simulink subsystem "PI_original"  (R2020b)
settings: Solver=VariableStepAuto  StartTime=0.0  StopTime=10.0  RelTol=1e-3
values from neighbouring files (symbols this model uses):
  Gamma12_z = -0.308384893038560    (= -0.308384893039)    [PI_original_parameters.m]
  Gamma21_z = -0.829434052560960    (= -0.829434052561)    [PI_original_parameters.m]
  K_P_11 = 1.653001431483017    (= 1.65300143148)    [PI_original_parameters.m]
  K_P_22 = 4.162509742530150    (= 4.16250974253)    [PI_original_parameters.m]
  T_I_11 = 841.6941455268073    (= 841.694145527)    [PI_original_parameters.m]
  T_I_22 = 757.1049307125121    (= 757.104930713)    [PI_original_parameters.m]
  zone_1_ctrl_idx = 5    [PI_original_parameters.m]
  zone_2_ctrl_idx = 10    [PI_original_parameters.m]
undefined symbols (not defined in the file or in its folder): T_c
settings Model: Creator=leop9  LastModifiedBy=Previ

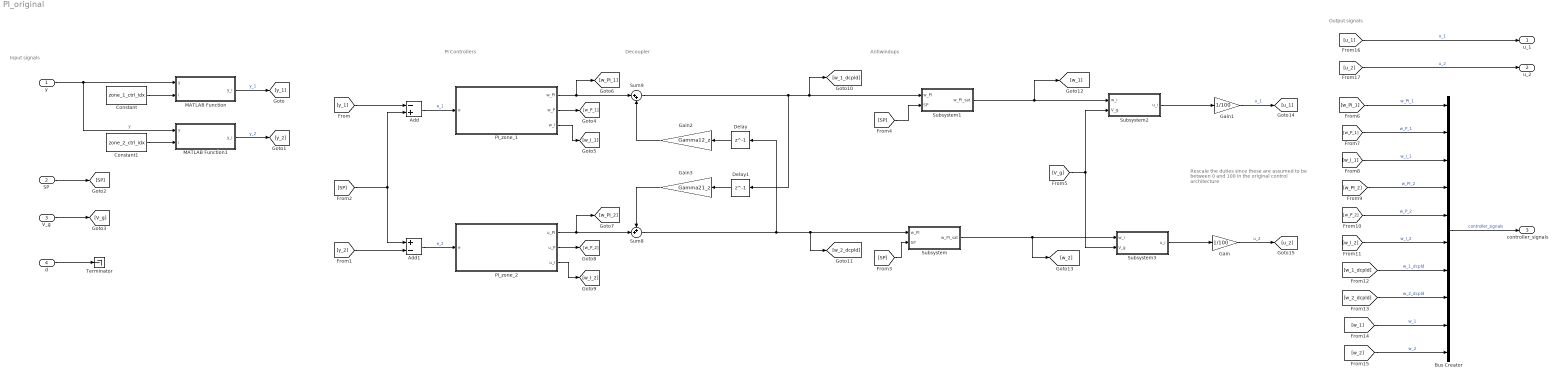
== system PI_original ==
  note: Output signals
  note: Antiwindups
  note: Decoupler
  note: Rescale the duties since these are assumed to be between 0 and 100 in the original control architecture
  note: PI Controllers
  note: Input signals
  y : Inport
  SP : Inport  Port=2
  V_g : Inport  Port=3
  d : Inport  Port=4
  Add : Sum  Inputs=-+
  Add1 : Sum  Inputs=+-
  Bus Creator : BusCreator  Inputs=10
  Constant : Constant  Value=zone_1_ctrl_idx
  Constant1 : Constant  Value=zone_2_ctrl_idx
  Delay : Delay  DelayLength=1  InitialCondition=0  SampleTime=T_c
  Delay1 : Delay  DelayLength=1  InitialCondition=0  SampleTime=T_c
  Gain : Gain  Gain=1/100
  Gain1 : Gain  Gain=1/100
  Gain2 : Gain  Gain=Gamma12_z
  Gain3 : Gain  Gain=Gamma21_z
  MATLAB Function : MATLAB Function  TreatAsAtomicUnit=on
  MATLAB Function1 : MATLAB Function  TreatAsAtomicUnit=on
  PI_zone_1 : Subsystem
  PI_zone_2 : Subsystem
  Subsystem : Subsystem
  Subsystem1 : Subsystem
  Subsystem2 : Subsystem
  Subsystem3 : Subsystem
  Sum8 : Sum  Inputs=++|
  Sum9 : Sum  Inputs=|++
  Terminator : Terminator
  u_1 : Outport
  u_2 : Outport  Port=2
  controller_signals : Outport  Port=3
  wires:
  Bus Creator/1 -> controller_signals/1  "controller_signals"
  [u_2] -> u_2/1  "u_2"
  [u_1] -> u_1/1  "u_1"
  [w_2] -> Bus Creator/10  "w_2"
  [w_1] -> Bus Creator/9  "w_1"
  [w_2_dcpld] -> Bus Creator/8  "w_2_dcpld"
  [w_1_dcpld] -> Bus Creator/7  "w_1_dcpld"
  [w_I_2] -> Bus Creator/6  "w_I_2"
  [w_P_2] -> Bus Creator/5  "w_P_2"
  [w_PI_2] -> Bus Creator/4  "w_PI_2"
  [w_I_1] -> Bus Creator/3  "w_I_1"
  [w_P_1] -> Bus Creator/2  "w_P_1"
  [w_PI_1] -> Bus Creator/1  "w_PI_1"
  PI_zone_2/3(u_I) -> [w_I_2]
  PI_zone_2/2(u_P) -> [w_P_2]
  PI_zone_1/3(w_I) -> [w_I_1]
  PI_zone_1/2(w_P) -> [w_P_1]
  [SP] -> Subsystem1/2(SP)
  [SP] -> Subsystem/2(SP)
  d/1 -> Terminator/1
  V_g/1 -> [V_g]
  SP/1 -> [SP]
  Constant1/1 -> MATLAB Function1/2(i)
  MATLAB Function1/1(y_i) -> [y_2]  "y_2"
  MATLAB Function/1(y_i) -> [y_1]  "y_1"
  Constant/1 -> MATLAB Function/2(i)
  y/1 -> MATLAB Function1/1(y), MATLAB Function/1(y)  "y"
  [y_2] -> Add1/2
  [y_1] -> Add/1
  Gain/1 -> [u_2]  "u_2"
  Gain1/1 -> [u_1]  "u_1"
  Subsystem2/1(u_i) -> Gain1/1
  Subsystem1/1(w_PI_sat) -> [w_1], Subsystem2/1(w_i)
  Subsystem3/1(u_i) -> Gain/1
  [V_g] -> Subsystem3/2(V_g), Subsystem2/2(V_g)
  [SP] -> Add1/1, Add/2
  Gain3/1 -> Sum8/1
  Add/1 -> PI_zone_1/1(e)  "e_1"
  Add1/1 -> PI_zone_2/1(e)  "e_2"
  Sum8/1 -> [w_2_dcpld], Subsystem/1(w_PI), Delay/1
  Sum9/1 -> Delay1/1, [w_1_dcpld], Subsystem1/1(w_PI)
  Subsystem/1(w_PI_sat) -> [w_2], Subsystem3/1(w_i)
  PI_zone_1/1(w_PI) -> [w_PI_1], Sum9/1
  PI_zone_2/1(u_PI) -> [w_PI_2], Sum8/2
  Gain2/1 -> Sum9/2
  Delay/1 -> Gain2/1
  Delay1/1 -> Gain3/1

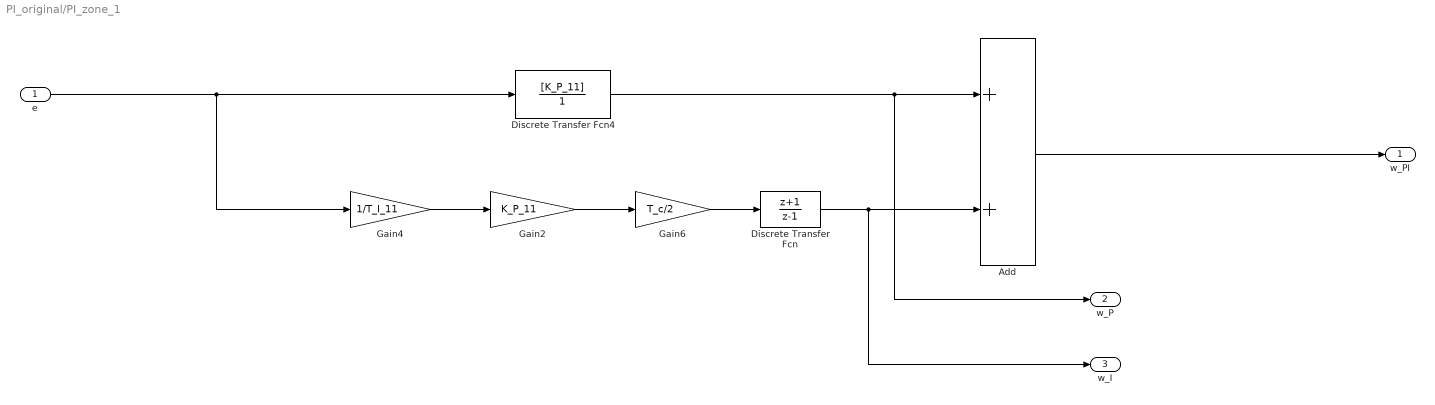
== system PI_original/PI_zone_1 ==
  e : Inport
  Add : Sum
  Discrete Transfer Fcn : DiscreteTransferFcn  Numerator=[1 1]  Denominator=[1 -1]  SampleTime=T_c
  Discrete Transfer Fcn4 : DiscreteTransferFcn  Numerator=[K_P_11]  Denominator=[1]  SampleTime=T_c
  Gain2 : Gain  Gain=K_P_11
  Gain4 : Gain  Gain=1/T_I_11
  Gain6 : Gain  Gain=T_c/2
  w_PI : Outport
  w_P : Outport  Port=2
  w_I : Outport  Port=3
  wires:
  Discrete Transfer Fcn4/1 -> Add/1, w_P/1
  Discrete Transfer Fcn/1 -> w_I/1, Add/2
  Gain2/1 -> Gain6/1
  Gain6/1 -> Discrete Transfer Fcn/1
  e/1 -> Discrete Transfer Fcn4/1, Gain4/1
  Add/1 -> w_PI/1
  Gain4/1 -> Gain2/1

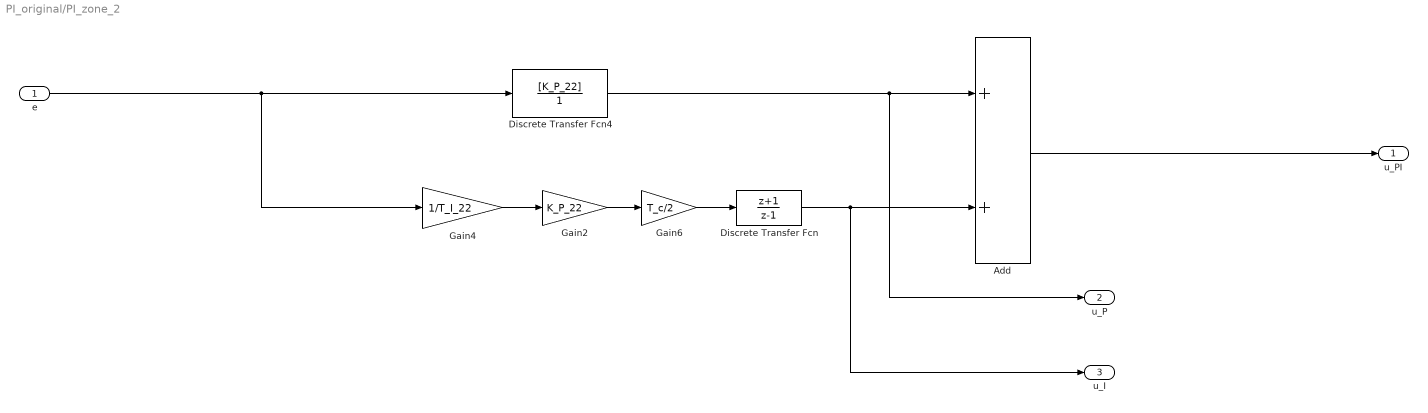
== system PI_original/PI_zone_2 ==
  e : Inport
  Add : Sum
  Discrete Transfer Fcn : DiscreteTransferFcn  Numerator=[1 1]  Denominator=[1 -1]  SampleTime=T_c
  Discrete Transfer Fcn4 : DiscreteTransferFcn  Numerator=[K_P_22]  Denominator=[1]  SampleTime=T_c
  Gain2 : Gain  Gain=K_P_22
  Gain4 : Gain  Gain=1/T_I_22
  Gain6 : Gain  Gain=T_c/2
  u_PI : Outport
  u_P : Outport  Port=2
  u_I : Outport  Port=3
  wires:
  Discrete Transfer Fcn4/1 -> Add/1, u_P/1
  Gain2/1 -> Gain6/1
  Gain6/1 -> Discrete Transfer Fcn/1
  Discrete Transfer Fcn/1 -> Add/2, u_I/1
  e/1 -> Discrete Transfer Fcn4/1, Gain4/1
  Add/1 -> u_PI/1
  Gain4/1 -> Gain2/1

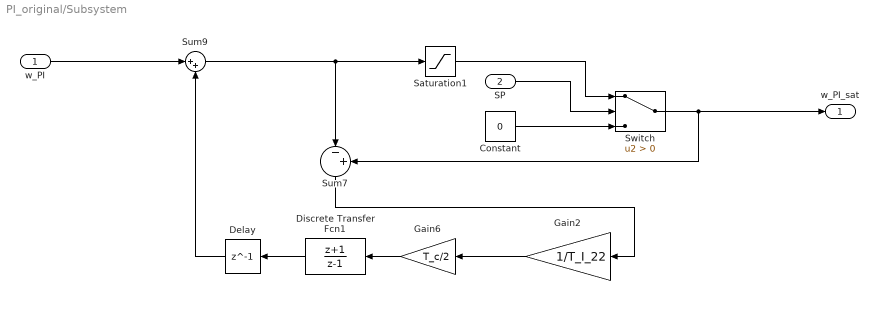
== system PI_original/Subsystem ==
  w_PI : Inport
  SP : Inport  Port=2
  Constant : Constant  Value=0
  Delay : Delay  DelayLength=1  InitialCondition=0  SampleTime=T_c
  Discrete Transfer Fcn1 : DiscreteTransferFcn  Numerator=[1 1]  Denominator=[1 -1]  SampleTime=T_c
  Gain2 : Gain  Gain=1/T_I_22
  Gain6 : Gain  Gain=T_c/2
  Saturation1 : Saturate  UpperLimit=100  LowerLimit=0
  Sum7 : Sum  Inputs=|-+
  Sum9 : Sum  Inputs=|++
  Switch : Switch  Criteria=u2 > Threshold
  w_PI_sat : Outport
  wires:
  Delay/1 -> Sum9/2
  Sum7/1 -> Gain2/1
  w_PI/1 -> Sum9/1
  SP/1 -> Switch/2
  Constant/1 -> Switch/3
  Saturation1/1 -> Switch/1
  Switch/1 -> Sum7/2, w_PI_sat/1
  Discrete Transfer Fcn1/1 -> Delay/1
  Gain2/1 -> Gain6/1
  Sum9/1 -> Saturation1/1, Sum7/1
  Gain6/1 -> Discrete Transfer Fcn1/1

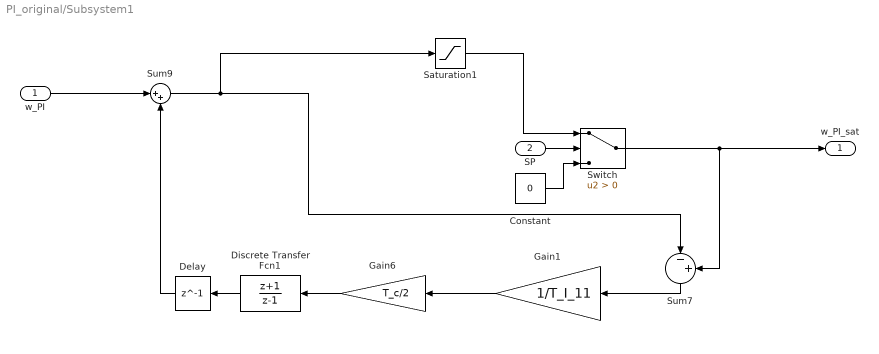
== system PI_original/Subsystem1 ==
  w_PI : Inport
  SP : Inport  Port=2
  Constant : Constant  Value=0
  Delay : Delay  DelayLength=1  InitialCondition=0  SampleTime=T_c
  Discrete Transfer Fcn1 : DiscreteTransferFcn  Numerator=[1 1]  Denominator=[1 -1]  SampleTime=T_c
  Gain1 : Gain  Gain=1/T_I_11
  Gain6 : Gain  Gain=T_c/2
  Saturation1 : Saturate  UpperLimit=100  LowerLimit=0
  Sum7 : Sum  Inputs=|-+
  Sum9 : Sum  Inputs=|++
  Switch : Switch  Criteria=u2 > Threshold
  w_PI_sat : Outport
  wires:
  Delay/1 -> Sum9/2
  Discrete Transfer Fcn1/1 -> Delay/1
  Constant/1 -> Switch/3
  Saturation1/1 -> Switch/1
  Sum7/1 -> Gain1/1
  Switch/1 -> Sum7/2, w_PI_sat/1
  Gain1/1 -> Gain6/1
  w_PI/1 -> Sum9/1
  Gain6/1 -> Discrete Transfer Fcn1/1
  Sum9/1 -> Sum7/1, Saturation1/1
  SP/1 -> Switch/2

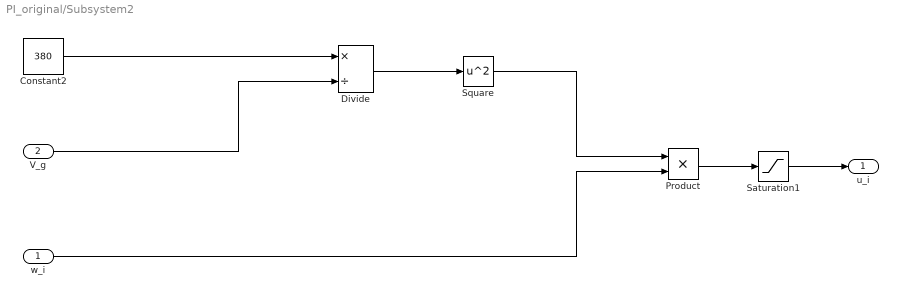
== system PI_original/Subsystem2 ==
  w_i : Inport
  V_g : Inport  Port=2
  Constant2 : Constant  Value=380
  Divide : Product  Inputs=*/  OutDataTypeStr=double  RndMeth=Nearest  LockScale=on
  Product : Product  OutDataTypeStr=double
  Saturation1 : Saturate  UpperLimit=100  LowerLimit=0
  Square : Math  Operator=square  OutDataTypeStr=double  RndMeth=Nearest
  u_i : Outport
  wires:
  Product/1 -> Saturation1/1
  w_i/1 -> Product/2
  V_g/1 -> Divide/2
  Square/1 -> Product/1
  Constant2/1 -> Divide/1
  Divide/1 -> Square/1
  Saturation1/1 -> u_i/1

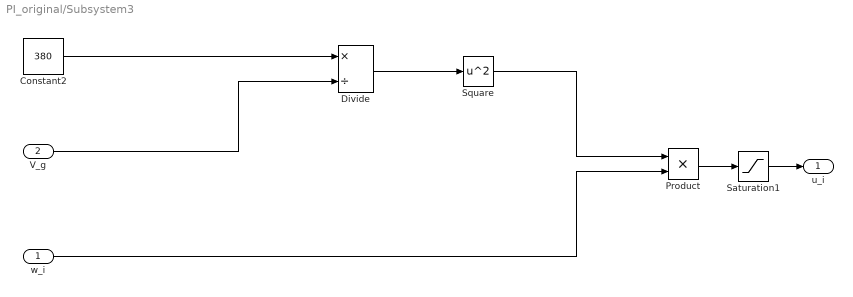
== system PI_original/Subsystem3 ==
  w_i : Inport
  V_g : Inport  Port=2
  Constant2 : Constant  Value=380
  Divide : Product  Inputs=*/  OutDataTypeStr=double  RndMeth=Nearest  LockScale=on
  Product : Product  OutDataTypeStr=double
  Saturation1 : Saturate  UpperLimit=100  LowerLimit=0
  Square : Math  Operator=square  OutDataTypeStr=double  RndMeth=Nearest
  u_i : Outport
  wires:
  Product/1 -> Saturation1/1
  w_i/1 -> Product/2
  V_g/1 -> Divide/2
  Square/1 -> Product/1
  Constant2/1 -> Divide/1
  Divide/1 -> Square/1
  Saturation1/1 -> u_i/1

== matlab function PI_original/MATLAB Function1 ==
  data: y input; y_i output; i input
function y_i = selectOutput(y, i)

y_i = y(i);

== matlab function PI_original/MATLAB Function ==
  data: y input; y_i output; i input
function y_i = selectOutput(y, i)

y_i = y(i);
